simulink model "pseudo_random_lut"  (R2020b)
settings: Solver=FixedStepDiscrete  StartTime=0.0  StopTime=stopTime  FixedStep=2.0833333333333333e-05  RelTol=1e-3
libraries: simulink x1
settings Model: Creator=Ross  LastModifiedBy=tyler
settings SolverCC: AutoInsertRateTranBlk=on
settings DataIOCC: SaveOutput=off  SaveTime=off  ReturnWorkspaceOutputs=off
settings OptimizationCC: BlockReduction=off  ConditionallyExecuteInputs=off  DefaultParameterBehavior=Inlined
settings DebuggingCC: ReadBeforeWriteMsg=DisableAll  WriteAfterWriteMsg=DisableAll  WriteAfterReadMsg=DisableAll  AlgebraicLoopMsg=error  MultiTaskDSMMsg=none  SingleTaskRateTransMsg=error  PregeneratedLibrarySubsystemCodeDiagnostic=none  ArithmeticOperatorsInVariantConditions=warning
settings HardwareCC: ProdBitPerPointer=32  ProdBitPerSizeT=32  ProdBitPerPtrDiffT=32  ProdLargestAtomicFloat=None  ProdIntDivRoundTo=Undefined  ProdEndianess=Unspecified  ProdWordSize=32  ProdHWDeviceType=ASIC/FPGA->ASIC/FPGA  TargetBitPerPointer=64  TargetBitPerSizeT=64  TargetBitPerPtrDiffT=64  TargetLongLongMode=on  TargetIntDivRoundTo=Zero  TargetEndianess=LittleEndian  TargetWordSize=64  TargetHWDeviceType=Custom Processor->MATLAB Host Computer  ProdEqTarget=off
settings ModelReferenceCC: UpdateModelReferenceTargets=IfOutOfDate
settings SFSimCC: SFSimEcho=off  SimUseLocalCustomCode=off  CustomCodeUndefinedFunction=UseInterfaceOnly
settings RTWCC: RTWUseLocalCustomCode=off

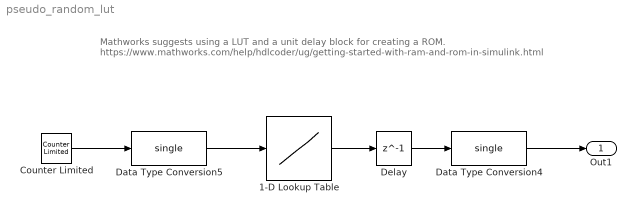
== system pseudo_random_lut ==
  note: Mathworks suggests using a LUT and a unit delay block for creating a ROM. https://www.mathworks.com/help/hdlcoder/ug/getting-started-with-ram-and-rom-in-simulink.html
  1-D Lookup Table : Lookup_n-D  NumberOfTableDimensions=1  BreakpointsForDimension1=[0:1023]  Table=rand(1,1024)  InternalRulePriority=Speed  RndMeth=Simplest  InputSameDT=on
  Counter Limited : simulink/Sources/Counter Limited  uplimit=1023  tsamp=mp.Ts_sim
  Data Type Conversion4 : DataTypeConversion  OutDataTypeStr=single
  Data Type Conversion5 : DataTypeConversion  OutDataTypeStr=single
  Delay : Delay  DelayLength=1
  Out1 : Outport  OutDataTypeStr=single  PortDimensions=1  SampleTime=[2.0833333333333333e-05,0]
  wires:
  Data Type Conversion5/1 -> 1-D Lookup Table/1
  1-D Lookup Table/1 -> Delay/1
  Counter Limited/1 -> Data Type Conversion5/1
  Data Type Conversion4/1 -> Out1/1
  Delay/1 -> Data Type Conversion4/1
